simulink model "Modular_Model_New_Board"  (R2016a)
settings: Solver=FixedStepAuto  SolverMode=SingleTasking  StartTime=0.0  StopTime=30e-3  FixedStep=SampleTime*1e-2  MinStep=SampleTime*1e-2  RelTol=1e-3
values from neighbouring files (symbols this model uses):
  ffund = 50    [sim_param_new_board.m]
  ModulationIndex1 = 0.9    [sim_param_new_board.m]
  ModulationIndex2 = 0.9    [sim_param_new_board.m]
  Module1Phase = 0    [sim_param_new_board.m]
  Module2Phase = 180    [sim_param_new_board.m]
  Rin = 10    [sim_param_new_board.m]
  Rload1 = Z1*PF    [sim_param_new_board.m]
  Rload2 = Z2*PF    [sim_param_new_board.m]
  Vmodule = 270    [sim_param_new_board.m]
  VpulseMax = 6    [sim_param_new_board.m]
  VpulseMin = -3    [sim_param_new_board.m]
libraries: elec_lib x139, fl_lib x67, nesl_utility x67, simulink x24, powerlib_meascontrol x4
(part 1 of 4)
settings Model: SimulationMode=accelerator  Creator=Furkan  LastModifiedBy=mesutto
settings DebuggingCC: SFUnexpectedBacktrackingDiag=error  SFNoUnconditionalDefaultTransitionDiag=error
settings GRTTargetCC: TargetLangStandard=C99 (ISO)  GeneratePreprocessorConditionals=Use local settings
settings ConfigComp: CovMetricSettings=dwe  CovHtmlReporting=off  CovSaveCumulativeToWorkspaceVar=off  CovSaveSingleToWorkspaceVar=off  CovExternalEMLEnable=on

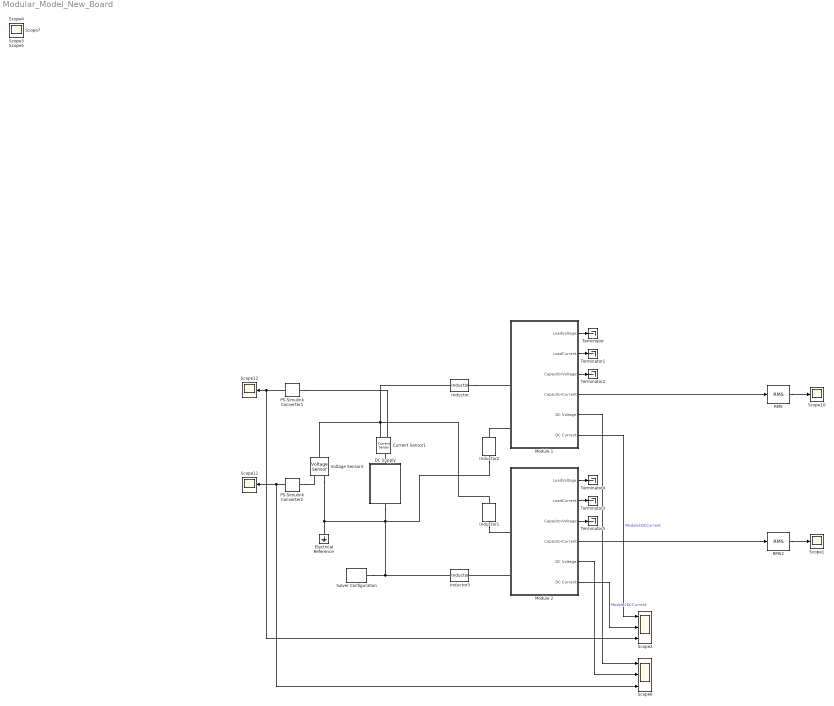
== system Modular_Model_New_Board ==
  Current Sensor1 : fl_lib/Electrical/Electrical Sensors/Current Sensor
  DC Supply : Subsystem
  Electrical Reference : fl_lib/Electrical/Electrical Elements/Electrical Reference
  Inductor : elec_lib/Passive Devices/Inductor  l=POS1 H  L_tol=20  enable_L_tol=0  tol_distribution=1  nSigma=4  r=0 Ohm  g=1e-9 1/Ohm  initI=0 A  enable_operating_limits=0  operating_limit_action=2  max_working_current=1 A  power_rating=1 W  enable_faults=0  fault_action=1  lambdaPercent=50  k_faulted=0.9999  turnsShort=0  openCct=0  groundShort=0  groundShortG=0 1/Ohm  tau_fault=1e-3 s  enable_temporal_fault=0  t_fault=1 s  enable_behavioral_fault=0  max_permissible_voltage=100 V  n_fail_on_voltage=1  max_permissible_current=1 A  t_fail_on_current=1 s
  Inductor1 : elec_lib/Passive Devices/Inductor  l=POS2 H  L_tol=20  enable_L_tol=0  tol_distribution=1  nSigma=4  r=0 Ohm  g=1e-9 1/Ohm  initI=0 A  enable_operating_limits=0  operating_limit_action=2  max_working_current=1 A  power_rating=1 W  enable_faults=0  fault_action=1  lambdaPercent=50  k_faulted=0.9999  turnsShort=0  openCct=0  groundShort=0  groundShortG=0 1/Ohm  tau_fault=1e-3 s  enable_temporal_fault=0  t_fault=1 s  enable_behavioral_fault=0  max_permissible_voltage=100 V  n_fail_on_voltage=1  max_permissible_current=1 A  t_fail_on_current=1 s
  Inductor2 : elec_lib/Passive Devices/Inductor  l=NEG1 H  L_tol=20  enable_L_tol=0  tol_distribution=1  nSigma=4  r=0 Ohm  g=1e-9 1/Ohm  initI=0 A  enable_operating_limits=0  operating_limit_action=2  max_working_current=1 A  power_rating=1 W  enable_faults=0  fault_action=1  lambdaPercent=50  k_faulted=0.9999  turnsShort=0  openCct=0  groundShort=0  groundShortG=0 1/Ohm  tau_fault=1e-3 s  enable_temporal_fault=0  t_fault=1 s  enable_behavioral_fault=0  max_permissible_voltage=100 V  n_fail_on_voltage=1  max_permissible_current=1 A  t_fail_on_current=1 s
  Inductor3 : elec_lib/Passive Devices/Inductor  l=NEG2 H  L_tol=20  enable_L_tol=0  tol_distribution=1  nSigma=4  r=0 Ohm  g=1e-9 1/Ohm  initI=0 A  enable_operating_limits=0  operating_limit_action=2  max_working_current=1 A  power_rating=1 W  enable_faults=0  fault_action=1  lambdaPercent=50  k_faulted=0.9999  turnsShort=0  openCct=0  groundShort=0  groundShortG=0 1/Ohm  tau_fault=1e-3 s  enable_temporal_fault=0  t_fault=1 s  enable_behavioral_fault=0  max_permissible_voltage=100 V  n_fail_on_voltage=1  max_permissible_current=1 A  t_fail_on_current=1 s
  Module 1 : Subsystem
  Module 2 : Subsystem
  PS-Simulink Converter1 : nesl_utility/PS-Simulink Converter  PhysicalDomain=network_engine_domain  SubClassName=ps_output  LeftPortType=input  RightPortType=output  PseudoPeriodic=off  Frequencies=[]  Unit=1  AffineConversion=off
  PS-Simulink Converter2 : nesl_utility/PS-Simulink Converter  PhysicalDomain=network_engine_domain  SubClassName=ps_output  LeftPortType=input  RightPortType=output  PseudoPeriodic=off  Frequencies=[]  Unit=1  AffineConversion=off
  RMS : powerlib_meascontrol/Measurements/RMS  TrueRMS=on  Freq=40000  RMSInit=0  Ts=0
  RMS2 : powerlib_meascontrol/Measurements/RMS  TrueRMS=on  Freq=40000  RMSInit=0  Ts=0
  Scope{1,3..5,7,10..12} (8 alike) : Scope
  Scope2 : Scope  NumInputPorts=3
  Scope6 : Scope  NumInputPorts=3
  Solver Configuration : nesl_utility/Solver Configuration  PhysicalDomain=network_engine_domain  SubClassName=solver  LeftPortType=input  RightPortType=generic  Accelerate=off  Tones=[]  Harmonics=[]  SimulateNoise=off  Profile=off  UseLocalSampling=off  EnableSwitchedLinearOptims=on  FrequencyDomain=off  UseCCode=off  RelTol=0.001  AbsTol=1e-06  MinStep=1e-09  ToWorkspace=off  RevertToSquareIcSolve=off  NumHomotopyIterations=100  PhasorMode=off  PhasorModeNumHarmonics=1  OverrideAbsTol=off  DoDC=off  ResidualTolerance=1e-09  UseLocalSolver=on  LocalSolverChoice=NE_BACKWARD_EULER_ADVANCER  LocalSolverSampleTime=SampleTime  DoFixedCost=on  MaxNonlinIter=3  MaxModeIter=2  LinearAlgebra=Sparse  DelaysMemoryBudget=1024  AutomaticFiltering=on  FilteringTimeConstant=0.001
  Terminator{,1..5} (6 alike) : Terminator
  Voltage Sensor3 : fl_lib/Electrical/Electrical Sensors/Voltage Sensor
  wires:
  Module 1/1(LoadVoltage) -> Terminator/1
  Module 1/4(CapacitorCurrent) -> RMS/1
  Module 2/1(LoadVoltage) -> Terminator4/1
  Module 2/4(CapacitorCurrent) -> RMS2/1
  PS-Simulink Converter2/1 -> Scope6/3, Scope11/1
  PS-Simulink Converter1/1 -> Scope12/1, Scope2/3
  RMS/1 -> Scope10/1
  Module 1/2(LoadCurrent) -> Terminator1/1
  Module 1/3(CapacitorVoltage) -> Terminator2/1
  Module 2/2(LoadCurrent) -> Terminator3/1
  Module 2/3(CapacitorVoltage) -> Terminator5/1
  RMS2/1 -> Scope1/1
  Module 1/6(DC Current) -> Scope2/1  "Module1DCCurrent"
  Module 2/6(DC Current) -> Scope2/2  "Module2DCCurrent"
  Module 1/5(DC Voltage) -> Scope6/1
  Module 2/5(DC Voltage) -> Scope6/2
  connections:
  Inductor1/RConn1 -- Inductor/LConn1 -- Current Sensor1/RConn2 -- Voltage Sensor3/LConn1
  Module 2/LConn3 -- Inductor3/RConn1
  Inductor/RConn1 -- Module 1/LConn2
  Module 1/LConn3 -- Inductor2/RConn1
  Inductor1/LConn1 -- Module 2/LConn2
  PS-Simulink Converter2/LConn1 -- Voltage Sensor3/RConn1
  Electrical Reference/LConn1 -- Inductor2/LConn1 -- DC Supply/LConn1 -- Inductor3/LConn1 -- Solver Configuration/RConn1 -- Voltage Sensor3/RConn2
  Current Sensor1/LConn1 -- DC Supply/RConn1
  PS-Simulink Converter1/LConn1 -- Current Sensor1/RConn1

== system Modular_Model_New_Board/DC Supply ==
  Inductor21 : elec_lib/Passive Devices/Inductor  l=Lin H  L_tol=20  enable_L_tol=0  tol_distribution=1  nSigma=4  r=0 Ohm  g=1e-9 1/Ohm  initI=0 A  enable_operating_limits=0  operating_limit_action=2  max_working_current=1 A  power_rating=1 W  enable_faults=0  fault_action=1  lambdaPercent=50  k_faulted=0.9999  turnsShort=0  openCct=0  groundShort=0  groundShortG=0 1/Ohm  tau_fault=1e-3 s  enable_temporal_fault=0  t_fault=1 s  enable_behavioral_fault=0  max_permissible_voltage=100 V  n_fail_on_voltage=1  max_permissible_current=1 A  t_fail_on_current=1 s
  Resistor18 : elec_lib/Passive Devices/Resistor  R=Rin Ohm  R_tol=5  enable_R_tol=0  tol_distribution=1  nSigma=4  enable_operating_limits=0  operating_limit_action=2  max_working_voltage=100 V  power_rating=1 W  enable_faults=0  fault_action=1  R_faulted=inf Ohm  enable_temporal_fault=0  t_fault=1 s  enable_behavioral_fault=0  max_permissible_current=1 A  t_fail_on_current=1 s  noise_mode=0  sample_time=1e-3 s  repeatability=1  auto_seed=728464307  user_seed=0  Tdevice=25 degC  alpha=3.93e-3 1/K  Tmeas=25 degC  thermal_mass=100 J/K  initial_temperature=25 degC  power_derating_T1=70 degC  power_derating_T2=155 degC  operating_temperature_range_vec=[-50, 150] degC
  Voltage Source : elec_lib/Sources/Voltage Source  dc_voltage=Vin V  ac_voltage=0 V  ac_shift=0 rad  ac_frequency=60 Hz  noise_mode=0  PSD=0 V^2/Hz  sample_time=1e-3 s  repeatability=1  auto_seed=1197368251  user_seed=0
  NEG : PMIOPort  Port=1  Side=Left
  POS : PMIOPort  Port=2  Side=Right
  connections:
  Resistor18/LConn1 -- Voltage Source/LConn1
  Voltage Source/RConn1 -- Inductor21/RConn1
  Inductor21/LConn1 -- NEG/RConn1
  Resistor18/RConn1 -- POS/RConn1

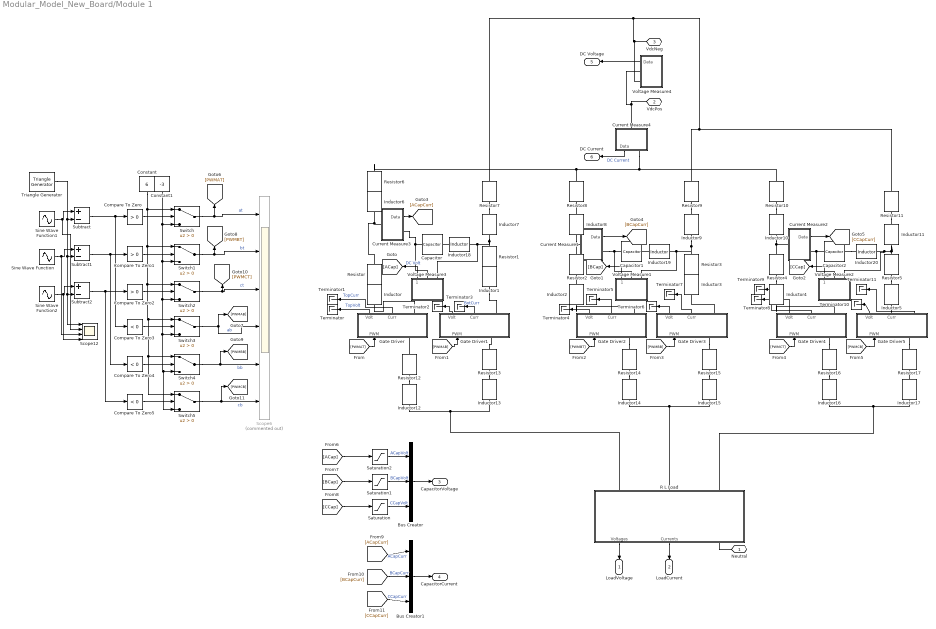
== system Modular_Model_New_Board/Module 1 ==
  Bus Creator : BusCreator  Inputs=3
  Bus Creator1 : BusCreator  Inputs=3
  Capacitor : elec_lib/Passive Devices/Capacitor  enable_table=0  c=C1A F  Cvec=[1e-05, 1e-06] F  Vvec=[0, 10] V  CV_table_symmetry=1  C_tol=0  enable_C_tol=0  tol_distribution=1  nSigma=4  r=21.1e-3 Ohm  g=0 1/Ohm  initV=0 V  enable_operating_limits=0  operating_limit_action=2  max_working_voltage_range=[-25, 25] V  power_rating=1 W  enable_faults=0  fault_action=1  Cscale_faulted=100  R_faulted=1e-3 Ohm  G_faulted=0 1/Ohm  tau_fault=1e-3 s  enable_temporal_fault=0  t_fault=1 s  enable_behavioral_fault=0  max_permissible_voltage_range=[-100, 100] V  t_fail_on_voltage=1 s
  Capacitor1 : elec_lib/Passive Devices/Capacitor  enable_table=0  c=C1B F  Cvec=[1e-05, 1e-06] F  Vvec=[0, 10] V  CV_table_symmetry=1  C_tol=0  enable_C_tol=0  tol_distribution=1  nSigma=4  r=21.1e-3 Ohm  g=0 1/Ohm  initV=0 V  enable_operating_limits=0  operating_limit_action=2  max_working_voltage_range=[-25, 25] V  power_rating=1 W  enable_faults=0  fault_action=1  Cscale_faulted=100  R_faulted=1e-3 Ohm  G_faulted=0 1/Ohm  tau_fault=1e-3 s  enable_temporal_fault=0  t_fault=1 s  enable_behavioral_fault=0  max_permissible_voltage_range=[-100, 100] V  t_fail_on_voltage=1 s
  Capacitor2 : elec_lib/Passive Devices/Capacitor  enable_table=0  c=C1C F  Cvec=[1e-05, 1e-06] F  Vvec=[0, 10] V  CV_table_symmetry=1  C_tol=0  enable_C_tol=0  tol_distribution=1  nSigma=4  r=21.1e-3 Ohm  g=0 1/Ohm  initV=0 V  enable_operating_limits=0  operating_limit_action=2  max_working_voltage_range=[-25, 25] V  power_rating=1 W  enable_faults=0  fault_action=1  Cscale_faulted=100  R_faulted=1e-3 Ohm  G_faulted=0 1/Ohm  tau_fault=1e-3 s  enable_temporal_fault=0  t_fault=1 s  enable_behavioral_fault=0  max_permissible_voltage_range=[-100, 100] V  t_fail_on_voltage=1 s
  Compare To Zero : simulink/Logic and Bit Operations/Compare To Zero  relop=>  OutDataTypeStr=boolean
  Compare To Zero1 : simulink/Logic and Bit Operations/Compare To Zero  relop=>  OutDataTypeStr=boolean
  Compare To Zero2 : simulink/Logic and Bit Operations/Compare To Zero  relop=>  OutDataTypeStr=boolean
  Compare To Zero3 : simulink/Logic and Bit Operations/Compare To Zero  relop=<  OutDataTypeStr=boolean
  Compare To Zero4 : simulink/Logic and Bit Operations/Compare To Zero  relop=<  OutDataTypeStr=boolean
  Compare To Zero5 : simulink/Logic and Bit Operations/Compare To Zero  relop=<  OutDataTypeStr=boolean
  Constant : Constant  Value=6
  Constant1 : Constant  Value=-3
  Current Measure1 : Subsystem
  Current Measure2 : Subsystem
  Current Measure3 : Subsystem
  Current Measure4 : Subsystem
  Gate Driver : Subsystem
  Gate Driver1 : Subsystem
  Gate Driver2 : Subsystem
  Gate Driver3 : Subsystem
  Gate Driver4 : Subsystem
  Gate Driver5 : Subsystem
  Inductor : elec_lib/Passive Devices/Inductor  l=ACapToDrain H  L_tol=20  enable_L_tol=0  tol_distribution=1  nSigma=4  r=0 Ohm  g=1e-9 1/Ohm  initI=0 A  enable_operating_limits=0  operating_limit_action=2  max_working_current=1 A  power_rating=1 W  enable_faults=0  fault_action=1  lambdaPercent=50  k_faulted=0.9999  turnsShort=0  openCct=0  groundShort=0  groundShortG=0 1/Ohm  tau_fault=1e-3 s  enable_temporal_fault=0  t_fault=1 s  enable_behavioral_fault=0  max_permissible_voltage=100 V  n_fail_on_voltage=1  max_permissible_current=1 A  t_fail_on_current=1 s
  Inductor1 : elec_lib/Passive Devices/Inductor  l=ACapToSource H  L_tol=20  enable_L_tol=0  tol_distribution=1  nSigma=4  r=0 Ohm  g=1e-9 1/Ohm  initI=0 A  enable_operating_limits=0  operating_limit_action=2  max_working_current=1 A  power_rating=1 W  enable_faults=0  fault_action=1  lambdaPercent=50  k_faulted=0.9999  turnsShort=0  openCct=0  groundShort=0  groundShortG=0 1/Ohm  tau_fault=1e-3 s  enable_temporal_fault=0  t_fault=1 s  enable_behavioral_fault=0  max_permissible_voltage=100 V  n_fail_on_voltage=1  max_permissible_current=1 A  t_fail_on_current=1 s
  Inductor10 : elec_lib/Passive Devices/Inductor  l=CPosToCap H  L_tol=20  enable_L_tol=0  tol_distribution=1  nSigma=4  r=0 Ohm  g=1e-9 1/Ohm  initI=0 A  enable_operating_limits=0  operating_limit_action=2  max_working_current=1 A  power_rating=1 W  enable_faults=0  fault_action=1  lambdaPercent=50  k_faulted=0.9999  turnsShort=0  openCct=0  groundShort=0  groundShortG=0 1/Ohm  tau_fault=1e-3 s  enable_temporal_fault=0  t_fault=1 s  enable_behavioral_fault=0  max_permissible_voltage=100 V  n_fail_on_voltage=1  max_permissible_current=1 A  t_fail_on_current=1 s
  Inductor11 : elec_lib/Passive Devices/Inductor  l=CNegToCap H  L_tol=20  enable_L_tol=0  tol_distribution=1  nSigma=4  r=0 Ohm  g=1e-9 1/Ohm  initI=0 A  enable_operating_limits=0  operating_limit_action=2  max_working_current=1 A  power_rating=1 W  enable_faults=0  fault_action=1  lambdaPercent=50  k_faulted=0.9999  turnsShort=0  openCct=0  groundShort=0  groundShortG=0 1/Ohm  tau_fault=1e-3 s  enable_temporal_fault=0  t_fault=1 s  enable_behavioral_fault=0  max_permissible_voltage=100 V  n_fail_on_voltage=1  max_permissible_current=1 A  t_fail_on_current=1 s
  Inductor12 : elec_lib/Passive Devices/Inductor  l=ASourceToLoad H  L_tol=20  enable_L_tol=0  tol_distribution=1  nSigma=4  r=0 Ohm  g=1e-9 1/Ohm  initI=0 A  enable_operating_limits=0  operating_limit_action=2  max_working_current=1 A  power_rating=1 W  enable_faults=0  fault_action=1  lambdaPercent=50  k_faulted=0.9999  turnsShort=0  openCct=0  groundShort=0  groundShortG=0 1/Ohm  tau_fault=1e-3 s  enable_temporal_fault=0  t_fault=1 s  enable_behavioral_fault=0  max_permissible_voltage=100 V  n_fail_on_voltage=1  max_permissible_current=1 A  t_fail_on_current=1 s
  Inductor13 : elec_lib/Passive Devices/Inductor  l=ADrainToLoad H  L_tol=20  enable_L_tol=0  tol_distribution=1  nSigma=4  r=0 Ohm  g=1e-9 1/Ohm  initI=0 A  enable_operating_limits=0  operating_limit_action=2  max_working_current=1 A  power_rating=1 W  enable_faults=0  fault_action=1  lambdaPercent=50  k_faulted=0.9999  turnsShort=0  openCct=0  groundShort=0  groundShortG=0 1/Ohm  tau_fault=1e-3 s  enable_temporal_fault=0  t_fault=1 s  enable_behavioral_fault=0  max_permissible_voltage=100 V  n_fail_on_voltage=1  max_permissible_current=1 A  t_fail_on_current=1 s
  Inductor14 : elec_lib/Passive Devices/Inductor  l=BSourceToLoad H  L_tol=20  enable_L_tol=0  tol_distribution=1  nSigma=4  r=0 Ohm  g=1e-9 1/Ohm  initI=0 A  enable_operating_limits=0  operating_limit_action=2  max_working_current=1 A  power_rating=1 W  enable_faults=0  fault_action=1  lambdaPercent=50  k_faulted=0.9999  turnsShort=0  openCct=0  groundShort=0  groundShortG=0 1/Ohm  tau_fault=1e-3 s  enable_temporal_fault=0  t_fault=1 s  enable_behavioral_fault=0  max_permissible_voltage=100 V  n_fail_on_voltage=1  max_permissible_current=1 A  t_fail_on_current=1 s
  Inductor15 : elec_lib/Passive Devices/Inductor  l=BDrainToLoad H  L_tol=20  enable_L_tol=0  tol_distribution=1  nSigma=4  r=0 Ohm  g=1e-9 1/Ohm  initI=0 A  enable_operating_limits=0  operating_limit_action=2  max_working_current=1 A  power_rating=1 W  enable_faults=0  fault_action=1  lambdaPercent=50  k_faulted=0.9999  turnsShort=0  openCct=0  groundShort=0  groundShortG=0 1/Ohm  tau_fault=1e-3 s  enable_temporal_fault=0  t_fault=1 s  enable_behavioral_fault=0  max_permissible_voltage=100 V  n_fail_on_voltage=1  max_permissible_current=1 A  t_fail_on_current=1 s
  Inductor16 : elec_lib/Passive Devices/Inductor  l=CSourceToLoad H  L_tol=20  enable_L_tol=0  tol_distribution=1  nSigma=4  r=0 Ohm  g=1e-9 1/Ohm  initI=0 A  enable_operating_limits=0  operating_limit_action=2  max_working_current=1 A  power_rating=1 W  enable_faults=0  fault_action=1  lambdaPercent=50  k_faulted=0.9999  turnsShort=0  openCct=0  groundShort=0  groundShortG=0 1/Ohm  tau_fault=1e-3 s  enable_temporal_fault=0  t_fault=1 s  enable_behavioral_fault=0  max_permissible_voltage=100 V  n_fail_on_voltage=1  max_permissible_current=1 A  t_fail_on_current=1 s
  Inductor17 : elec_lib/Passive Devices/Inductor  l=CDrainToLoad H  L_tol=20  enable_L_tol=0  tol_distribution=1  nSigma=4  r=0 Ohm  g=1e-9 1/Ohm  initI=0 A  enable_operating_limits=0  operating_limit_action=2  max_working_current=1 A  power_rating=1 W  enable_faults=0  fault_action=1  lambdaPercent=50  k_faulted=0.9999  turnsShort=0  openCct=0  groundShort=0  groundShortG=0 1/Ohm  tau_fault=1e-3 s  enable_temporal_fault=0  t_fault=1 s  enable_behavioral_fault=0  max_permissible_voltage=100 V  n_fail_on_voltage=1  max_permissible_current=1 A  t_fail_on_current=1 s
  Inductor18 : elec_lib/Passive Devices/Inductor  l=19e-9 H  L_tol=20  enable_L_tol=0  tol_distribution=1  nSigma=4  r=0 Ohm  g=1e-9 1/Ohm  initI=0 A  enable_operating_limits=0  operating_limit_action=2  max_working_current=1 A  power_rating=1 W  enable_faults=0  fault_action=1  lambdaPercent=50  k_faulted=0.9999  turnsShort=0  openCct=0  groundShort=0  groundShortG=0 1/Ohm  tau_fault=1e-3 s  enable_temporal_fault=0  t_fault=1 s  enable_behavioral_fault=0  max_permissible_voltage=100 V  n_fail_on_voltage=1  max_permissible_current=1 A  t_fail_on_current=1 s
  Inductor19 : elec_lib/Passive Devices/Inductor  l=19e-9 H  L_tol=20  enable_L_tol=0  tol_distribution=1  nSigma=4  r=0 Ohm  g=1e-9 1/Ohm  initI=0 A  enable_operating_limits=0  operating_limit_action=2  max_working_current=1 A  power_rating=1 W  enable_faults=0  fault_action=1  lambdaPercent=50  k_faulted=0.9999  turnsShort=0  openCct=0  groundShort=0  groundShortG=0 1/Ohm  tau_fault=1e-3 s  enable_temporal_fault=0  t_fault=1 s  enable_behavioral_fault=0  max_permissible_voltage=100 V  n_fail_on_voltage=1  max_permissible_current=1 A  t_fail_on_current=1 s
  Inductor2 : elec_lib/Passive Devices/Inductor  l=BCapToDrain H  L_tol=20  enable_L_tol=0  tol_distribution=1  nSigma=4  r=0 Ohm  g=1e-9 1/Ohm  initI=0 A  enable_operating_limits=0  operating_limit_action=2  max_working_current=1 A  power_rating=1 W  enable_faults=0  fault_action=1  lambdaPercent=50  k_faulted=0.9999  turnsShort=0  openCct=0  groundShort=0  groundShortG=0 1/Ohm  tau_fault=1e-3 s  enable_temporal_fault=0  t_fault=1 s  enable_behavioral_fault=0  max_permissible_voltage=100 V  n_fail_on_voltage=1  max_permissible_current=1 A  t_fail_on_current=1 s
  Inductor20 : elec_lib/Passive Devices/Inductor  l=19e-9 H  L_tol=20  enable_L_tol=0  tol_distribution=1  nSigma=4  r=0 Ohm  g=1e-9 1/Ohm  initI=0 A  enable_operating_limits=0  operating_limit_action=2  max_working_current=1 A  power_rating=1 W  enable_faults=0  fault_action=1  lambdaPercent=50  k_faulted=0.9999  turnsShort=0  openCct=0  groundShort=0  groundShortG=0 1/Ohm  tau_fault=1e-3 s  enable_temporal_fault=0  t_fault=1 s  enable_behavioral_fault=0  max_permissible_voltage=100 V  n_fail_on_voltage=1  max_permissible_current=1 A  t_fail_on_current=1 s
  Inductor3 : elec_lib/Passive Devices/Inductor  l=BCapToSource H  L_tol=20  enable_L_tol=0  tol_distribution=1  nSigma=4  r=0 Ohm  g=1e-9 1/Ohm  initI=0 A  enable_operating_limits=0  operating_limit_action=2  max_working_current=1 A  power_rating=1 W  enable_faults=0  fault_action=1  lambdaPercent=50  k_faulted=0.9999  turnsShort=0  openCct=0  groundShort=0  groundShortG=0 1/Ohm  tau_fault=1e-3 s  enable_temporal_fault=0  t_fault=1 s  enable_behavioral_fault=0  max_permissible_voltage=100 V  n_fail_on_voltage=1  max_permissible_current=1 A  t_fail_on_current=1 s
  Inductor4 : elec_lib/Passive Devices/Inductor  l=CCapToDrain H  L_tol=20  enable_L_tol=0  tol_distribution=1  nSigma=4  r=0 Ohm  g=1e-9 1/Ohm  initI=0 A  enable_operating_limits=0  operating_limit_action=2  max_working_current=1 A  power_rating=1 W  enable_faults=0  fault_action=1  lambdaPercent=50  k_faulted=0.9999  turnsShort=0  openCct=0  groundShort=0  groundShortG=0 1/Ohm  tau_fault=1e-3 s  enable_temporal_fault=0  t_fault=1 s  enable_behavioral_fault=0  max_permissible_voltage=100 V  n_fail_on_voltage=1  max_permissible_current=1 A  t_fail_on_current=1 s
  Inductor5 : elec_lib/Passive Devices/Inductor  l=CCapToSource H  L_tol=20  enable_L_tol=0  tol_distribution=1  nSigma=4  r=0 Ohm  g=1e-9 1/Ohm  initI=0 A  enable_operating_limits=0  operating_limit_action=2  max_working_current=1 A  power_rating=1 W  enable_faults=0  fault_action=1  lambdaPercent=50  k_faulted=0.9999  turnsShort=0  openCct=0  groundShort=0  groundShortG=0 1/Ohm  tau_fault=1e-3 s  enable_temporal_fault=0  t_fault=1 s  enable_behavioral_fault=0  max_permissible_voltage=100 V  n_fail_on_voltage=1  max_permissible_current=1 A  t_fail_on_current=1 s
  Inductor6 : elec_lib/Passive Devices/Inductor  l=APosToCap H  L_tol=20  enable_L_tol=0  tol_distribution=1  nSigma=4  r=0 Ohm  g=1e-9 1/Ohm  initI=0 A  enable_operating_limits=0  operating_limit_action=2  max_working_current=1 A  power_rating=1 W  enable_faults=0  fault_action=1  lambdaPercent=50  k_faulted=0.9999  turnsShort=0  openCct=0  groundShort=0  groundShortG=0 1/Ohm  tau_fault=1e-3 s  enable_temporal_fault=0  t_fault=1 s  enable_behavioral_fault=0  max_permissible_voltage=100 V  n_fail_on_voltage=1  max_permissible_current=1 A  t_fail_on_current=1 s
  Inductor7 : elec_lib/Passive Devices/Inductor  l=ANegToCap H  L_tol=20  enable_L_tol=0  tol_distribution=1  nSigma=4  r=0 Ohm  g=1e-9 1/Ohm  initI=0 A  enable_operating_limits=0  operating_limit_action=2  max_working_current=1 A  power_rating=1 W  enable_faults=0  fault_action=1  lambdaPercent=50  k_faulted=0.9999  turnsShort=0  openCct=0  groundShort=0  groundShortG=0 1/Ohm  tau_fault=1e-3 s  enable_temporal_fault=0  t_fault=1 s  enable_behavioral_fault=0  max_permissible_voltage=100 V  n_fail_on_voltage=1  max_permissible_current=1 A  t_fail_on_current=1 s
  Inductor8 : elec_lib/Passive Devices/Inductor  l=BPosToCap H  L_tol=20  enable_L_tol=0  tol_distribution=1  nSigma=4  r=0 Ohm  g=1e-9 1/Ohm  initI=0 A  enable_operating_limits=0  operating_limit_action=2  max_working_current=1 A  power_rating=1 W  enable_faults=0  fault_action=1  lambdaPercent=50  k_faulted=0.9999  turnsShort=0  openCct=0  groundShort=0  groundShortG=0 1/Ohm  tau_fault=1e-3 s  enable_temporal_fault=0  t_fault=1 s  enable_behavioral_fault=0  max_permissible_voltage=100 V  n_fail_on_voltage=1  max_permissible_current=1 A  t_fail_on_current=1 s
  Inductor9 : elec_lib/Passive Devices/Inductor  l=BNegToCap H  L_tol=20  enable_L_tol=0  tol_distribution=1  nSigma=4  r=0 Ohm  g=1e-9 1/Ohm  initI=0 A  enable_operating_limits=0  operating_limit_action=2  max_working_current=1 A  power_rating=1 W  enable_faults=0  fault_action=1  lambdaPercent=50  k_faulted=0.9999  turnsShort=0  openCct=0  groundShort=0  groundShortG=0 1/Ohm  tau_fault=1e-3 s  enable_temporal_fault=0  t_fault=1 s  enable_behavioral_fault=0  max_permissible_voltage=100 V  n_fail_on_voltage=1  max_permissible_current=1 A  t_fail_on_current=1 s
  R L Load : Subsystem
  Resistor : elec_lib/Passive Devices/Resistor  R=854e-6 Ohm  R_tol=5  enable_R_tol=0  tol_distribution=1  nSigma=4  enable_operating_limits=0  operating_limit_action=2  max_working_voltage=100 V  power_rating=1 W  enable_faults=0  fault_action=1  R_faulted=inf Ohm  enable_temporal_fault=0  t_fault=1 s  enable_behavioral_fault=0  max_permissible_current=1 A  t_fail_on_current=1 s  noise_mode=0  sample_time=1e-3 s  repeatability=1  auto_seed=1725752364  user_seed=0  Tdevice=25 degC  alpha=3.93e-3 1/K  Tmeas=25 degC  thermal_mass=100 J/K  initial_temperature=25 degC  power_derating_T1=70 degC  power_derating_T2=155 degC  operating_temperature_range_vec=[-50, 150] degC
  Resistor1 : elec_lib/Passive Devices/Resistor  R=664e-6 Ohm  R_tol=5  enable_R_tol=0  tol_distribution=1  nSigma=4  enable_operating_limits=0  operating_limit_action=2  max_working_voltage=100 V  power_rating=1 W  enable_faults=0  fault_action=1  R_faulted=inf Ohm  enable_temporal_fault=0  t_fault=1 s  enable_behavioral_fault=0  max_permissible_current=1 A  t_fail_on_current=1 s  noise_mode=0  sample_time=1e-3 s  repeatability=1  auto_seed=1978802833  user_seed=0  Tdevice=25 degC  alpha=3.93e-3 1/K  Tmeas=25 degC  thermal_mass=100 J/K  initial_temperature=25 degC  power_derating_T1=70 degC  power_derating_T2=155 degC  operating_temperature_range_vec=[-50, 150] degC
  Resistor10 : elec_lib/Passive Devices/Resistor  R=867e-6 Ohm  R_tol=5  enable_R_tol=0  tol_distribution=1  nSigma=4  enable_operating_limits=0  operating_limit_action=2  max_working_voltage=100 V  power_rating=1 W  enable_faults=0  fault_action=1  R_faulted=inf Ohm  enable_temporal_fault=0  t_fault=1 s  enable_behavioral_fault=0  max_permissible_current=1 A  t_fail_on_current=1 s  noise_mode=0  sample_time=1e-3 s  repeatability=1  auto_seed=3085328168  user_seed=0  Tdevice=25 degC  alpha=3.93e-3 1/K  Tmeas=25 degC  thermal_mass=100 J/K  initial_temperature=25 degC  power_derating_T1=70 degC  power_derating_T2=155 degC  operating_temperature_range_vec=[-50, 150] degC
  Resistor11 : elec_lib/Passive Devices/Resistor  R=595e-6 Ohm  R_tol=5  enable_R_tol=0  tol_distribution=1  nSigma=4  enable_operating_limits=0  operating_limit_action=2  max_working_voltage=100 V  power_rating=1 W  enable_faults=0  fault_action=1  R_faulted=inf Ohm  enable_temporal_fault=0  t_fault=1 s  enable_behavioral_fault=0  max_permissible_current=1 A  t_fail_on_current=1 s  noise_mode=0  sample_time=1e-3 s  repeatability=1  auto_seed=4160317194  user_seed=0  Tdevice=25 degC  alpha=3.93e-3 1/K  Tmeas=25 degC  thermal_mass=100 J/K  initial_temperature=25 degC  power_derating_T1=70 degC  power_derating_T2=155 degC  operating_temperature_range_vec=[-50, 150] degC
  Resistor12 : elec_lib/Passive Devices/Resistor  R=218.8e-6 Ohm  R_tol=5  enable_R_tol=0  tol_distribution=1  nSigma=4  enable_operating_limits=0  operating_limit_action=2  max_working_voltage=100 V  power_rating=1 W  enable_faults=0  fault_action=1  R_faulted=inf Ohm  enable_temporal_fault=0  t_fault=1 s  enable_behavioral_fault=0  max_permissible_current=1 A  t_fail_on_current=1 s  noise_mode=0  sample_time=1e-3 s  repeatability=1  auto_seed=1396490070  user_seed=0  Tdevice=25 degC  alpha=3.93e-3 1/K  Tmeas=25 degC  thermal_mass=100 J/K  initial_temperature=25 degC  power_derating_T1=70 degC  power_derating_T2=155 degC  operating_temperature_range_vec=[-50, 150] degC
  Resistor13 : elec_lib/Passive Devices/Resistor  R=218.8e-6 Ohm  R_tol=5  enable_R_tol=0  tol_distribution=1  nSigma=4  enable_operating_limits=0  operating_limit_action=2  max_working_voltage=100 V  power_rating=1 W  enable_faults=0  fault_action=1  R_faulted=inf Ohm  enable_temporal_fault=0  t_fault=1 s  enable_behavioral_fault=0  max_permissible_current=1 A  t_fail_on_current=1 s  noise_mode=0  sample_time=1e-3 s  repeatability=1  auto_seed=453673974  user_seed=0  Tdevice=25 degC  alpha=3.93e-3 1/K  Tmeas=25 degC  thermal_mass=100 J/K  initial_temperature=25 degC  power_derating_T1=70 degC  power_derating_T2=155 degC  operating_temperature_range_vec=[-50, 150] degC
  Resistor14 : elec_lib/Passive Devices/Resistor  R=218e-6 Ohm  R_tol=5  enable_R_tol=0  tol_distribution=1  nSigma=4  enable_operating_limits=0  operating_limit_action=2  max_working_voltage=100 V  power_rating=1 W  enable_faults=0  fault_action=1  R_faulted=inf Ohm  enable_temporal_fault=0  t_fault=1 s  enable_behavioral_fault=0  max_permissible_current=1 A  t_fail_on_current=1 s  noise_mode=0  sample_time=1e-3 s  repeatability=1  auto_seed=2624047458  user_seed=0  Tdevice=25 degC  alpha=3.93e-3 1/K  Tmeas=25 degC  thermal_mass=100 J/K  initial_temperature=25 degC  power_derating_T1=70 degC  power_derating_T2=155 degC  operating_temperature_range_vec=[-50, 150] degC
  Resistor15 : elec_lib/Passive Devices/Resistor  R=218e-6 Ohm  R_tol=5  enable_R_tol=0  tol_distribution=1  nSigma=4  enable_operating_limits=0  operating_limit_action=2  max_working_voltage=100 V  power_rating=1 W  enable_faults=0  fault_action=1  R_faulted=inf Ohm  enable_temporal_fault=0  t_fault=1 s  enable_behavioral_fault=0  max_permissible_current=1 A  t_fail_on_current=1 s  noise_mode=0  sample_time=1e-3 s  repeatability=1  auto_seed=3344930158  user_seed=0  Tdevice=25 degC  alpha=3.93e-3 1/K  Tmeas=25 degC  thermal_mass=100 J/K  initial_temperature=25 degC  power_derating_T1=70 degC  power_derating_T2=155 degC  operating_temperature_range_vec=[-50, 150] degC
  Resistor16 : elec_lib/Passive Devices/Resistor  R=218.3e-6 Ohm  R_tol=5  enable_R_tol=0  tol_distribution=1  nSigma=4  enable_operating_limits=0  operating_limit_action=2  max_working_voltage=100 V  power_rating=1 W  enable_faults=0  fault_action=1  R_faulted=inf Ohm  enable_temporal_fault=0  t_fault=1 s  enable_behavioral_fault=0  max_permissible_current=1 A  t_fail_on_current=1 s  noise_mode=0  sample_time=1e-3 s  repeatability=1  auto_seed=1818716438  user_seed=0  Tdevice=25 degC  alpha=3.93e-3 1/K  Tmeas=25 degC  thermal_mass=100 J/K  initial_temperature=25 degC  power_derating_T1=70 degC  power_derating_T2=155 degC  operating_temperature_range_vec=[-50, 150] degC
  Resistor17 : elec_lib/Passive Devices/Resistor  R=218.3e-6 Ohm  R_tol=5  enable_R_tol=0  tol_distribution=1  nSigma=4  enable_operating_limits=0  operating_limit_action=2  max_working_voltage=100 V  power_rating=1 W  enable_faults=0  fault_action=1  R_faulted=inf Ohm  enable_temporal_fault=0  t_fault=1 s  enable_behavioral_fault=0  max_permissible_current=1 A  t_fail_on_current=1 s  noise_mode=0  sample_time=1e-3 s  repeatability=1  auto_seed=390083043  user_seed=0  Tdevice=25 degC  alpha=3.93e-3 1/K  Tmeas=25 degC  thermal_mass=100 J/K  initial_temperature=25 degC  power_derating_T1=70 degC  power_derating_T2=155 degC  operating_temperature_range_vec=[-50, 150] degC
  Resistor2 : elec_lib/Passive Devices/Resistor  R=813e-6 Ohm  R_tol=5  enable_R_tol=0  tol_distribution=1  nSigma=4  enable_operating_limits=0  operating_limit_action=2  max_working_voltage=100 V  power_rating=1 W  enable_faults=0  fault_action=1  R_faulted=inf Ohm  enable_temporal_fault=0  t_fault=1 s  enable_behavioral_fault=0  max_permissible_current=1 A  t_fail_on_current=1 s  noise_mode=0  sample_time=1e-3 s  repeatability=1  auto_seed=4216102895  user_seed=0  Tdevice=25 degC  alpha=3.93e-3 1/K  Tmeas=25 degC  thermal_mass=100 J/K  initial_temperature=25 degC  power_derating_T1=70 degC  power_derating_T2=155 degC  operating_temperature_range_vec=[-50, 150] degC
  Resistor3 : elec_lib/Passive Devices/Resistor  R=664e-6 Ohm  R_tol=5  enable_R_tol=0  tol_distribution=1  nSigma=4  enable_operating_limits=0  operating_limit_action=2  max_working_voltage=100 V  power_rating=1 W  enable_faults=0  fault_action=1  R_faulted=inf Ohm  enable_temporal_fault=0  t_fault=1 s  enable_behavioral_fault=0  max_permissible_current=1 A  t_fail_on_current=1 s  noise_mode=0  sample_time=1e-3 s  repeatability=1  auto_seed=671754155  user_seed=0  Tdevice=25 degC  alpha=3.93e-3 1/K  Tmeas=25 degC  thermal_mass=100 J/K  initial_temperature=25 degC  power_derating_T1=70 degC  power_derating_T2=155 degC  operating_temperature_range_vec=[-50, 150] degC
  Resistor4 : elec_lib/Passive Devices/Resistor  R=854e-6 Ohm  R_tol=5  enable_R_tol=0  tol_distribution=1  nSigma=4  enable_operating_limits=0  operating_limit_action=2  max_working_voltage=100 V  power_rating=1 W  enable_faults=0  fault_action=1  R_faulted=inf Ohm  enable_temporal_fault=0  t_fault=1 s  enable_behavioral_fault=0  max_permissible_current=1 A  t_fail_on_current=1 s  noise_mode=0  sample_time=1e-3 s  repeatability=1  auto_seed=3674442472  user_seed=0  Tdevice=25 degC  alpha=3.93e-3 1/K  Tmeas=25 degC  thermal_mass=100 J/K  initial_temperature=25 degC  power_derating_T1=70 degC  power_derating_T2=155 degC  operating_temperature_range_vec=[-50, 150] degC
  Resistor5 : elec_lib/Passive Devices/Resistor  R=664e-6 Ohm  R_tol=5  enable_R_tol=0  tol_distribution=1  nSigma=4  enable_operating_limits=0  operating_limit_action=2  max_working_voltage=100 V  power_rating=1 W  enable_faults=0  fault_action=1  R_faulted=inf Ohm  enable_temporal_fault=0  t_fault=1 s  enable_behavioral_fault=0  max_permissible_current=1 A  t_fail_on_current=1 s  noise_mode=0  sample_time=1e-3 s  repeatability=1  auto_seed=2769242599  user_seed=0  Tdevice=25 degC  alpha=3.93e-3 1/K  Tmeas=25 degC  thermal_mass=100 J/K  initial_temperature=25 degC  power_derating_T1=70 degC  power_derating_T2=155 degC  operating_temperature_range_vec=[-50, 150] degC
  Resistor6 : elec_lib/Passive Devices/Resistor  R=1037e-6 Ohm  R_tol=5  enable_R_tol=0  tol_distribution=1  nSigma=4  enable_operating_limits=0  operating_limit_action=2  max_working_voltage=100 V  power_rating=1 W  enable_faults=0  fault_action=1  R_faulted=inf Ohm  enable_temporal_fault=0  t_fault=1 s  enable_behavioral_fault=0  max_permissible_current=1 A  t_fail_on_current=1 s  noise_mode=0  sample_time=1e-3 s  repeatability=1  auto_seed=2280044724  user_seed=0  Tdevice=25 degC  alpha=3.93e-3 1/K  Tmeas=25 degC  thermal_mass=100 J/K  initial_temperature=25 degC  power_derating_T1=70 degC  power_derating_T2=155 degC  operating_temperature_range_vec=[-50, 150] degC
  Resistor7 : elec_lib/Passive Devices/Resistor  R=1422e-6 Ohm  R_tol=5  enable_R_tol=0  tol_distribution=1  nSigma=4  enable_operating_limits=0  operating_limit_action=2  max_working_voltage=100 V  power_rating=1 W  enable_faults=0  fault_action=1  R_faulted=inf Ohm  enable_temporal_fault=0  t_fault=1 s  enable_behavioral_fault=0  max_permissible_current=1 A  t_fail_on_current=1 s  noise_mode=0  sample_time=1e-3 s  repeatability=1  auto_seed=2810822912  user_seed=0  Tdevice=25 degC  alpha=3.93e-3 1/K  Tmeas=25 degC  thermal_mass=100 J/K  initial_temperature=25 degC  power_derating_T1=70 degC  power_derating_T2=155 degC  operating_temperature_range_vec=[-50, 150] degC
  Resistor8 : elec_lib/Passive Devices/Resistor  R=611e-6 Ohm  R_tol=5  enable_R_tol=0  tol_distribution=1  nSigma=4  enable_operating_limits=0  operating_limit_action=2  max_working_voltage=100 V  power_rating=1 W  enable_faults=0  fault_action=1  R_faulted=inf Ohm  enable_temporal_fault=0  t_fault=1 s  enable_behavioral_fault=0  max_permissible_current=1 A  t_fail_on_current=1 s  noise_mode=0  sample_time=1e-3 s  repeatability=1  auto_seed=1750711121  user_seed=0  Tdevice=25 degC  alpha=3.93e-3 1/K  Tmeas=25 degC  thermal_mass=100 J/K  initial_temperature=25 degC  power_derating_T1=70 degC  power_derating_T2=155 degC  operating_temperature_range_vec=[-50, 150] degC
  Resistor9 : elec_lib/Passive Devices/Resistor  R=662e-6 Ohm  R_tol=5  enable_R_tol=0  tol_distribution=1  nSigma=4  enable_operating_limits=0  operating_limit_action=2  max_working_voltage=100 V  power_rating=1 W  enable_faults=0  fault_action=1  R_faulted=inf Ohm  enable_temporal_fault=0  t_fault=1 s  enable_behavioral_fault=0  max_permissible_current=1 A  t_fail_on_current=1 s  noise_mode=0  sample_time=1e-3 s  repeatability=1  auto_seed=3521792535  user_seed=0  Tdevice=25 degC  alpha=3.93e-3 1/K  Tmeas=25 degC  thermal_mass=100 J/K  initial_temperature=25 degC  power_derating_T1=70 degC  power_derating_T2=155 degC  operating_temperature_range_vec=[-50, 150] degC
  Saturation : Saturate  UpperLimit=Vmodule*1.5  LowerLimit=-20
  Saturation1 : Saturate  UpperLimit=Vmodule*1.5  LowerLimit=-20
  Saturation2 : Saturate  UpperLimit=Vmodule*1.5  LowerLimit=-20
  Scope12 : Scope  NumInputPorts=4
  Scope6 : Scope  Commented=on  NumInputPorts=6
  Sine Wave Function : Sin  Amplitude=ModulationIndex1  Frequency=ffund*2*pi  Phase=-2*pi/3  SampleTime=0
  Sine Wave Function1 : Sin  Amplitude=ModulationIndex1  Frequency=ffund*2*pi  SampleTime=0
  Sine Wave Function2 : Sin  Amplitude=ModulationIndex1  Frequency=ffund*2*pi  Phase=2*pi/3  SampleTime=0
  Subtract : Sum  Inputs=+-
  Subtract1 : Sum  Inputs=+-
  Subtract2 : Sum  Inputs=+-
  Switch{,1..5} (6 alike) : Switch  Criteria=u2 > Threshold
  Terminator{,1..11} (12 alike) : Terminator
  Triangle Generator : powerlib_meascontrol/Pulse & Signal Generators/Triangle Generator  Freq=fsw  Phase=Module1Phase  Ts=0
  Voltage Measure1 : Subsystem
  Voltage Measure2 : Subsystem
  Voltage Measure3 : Subsystem
  Voltage Measure4 : Subsystem
  "Neutral " : PMIOPort  Port=1  Side=Left
  VdcPos : PMIOPort  Port=2  Side=Left
  VdcNeg : PMIOPort  Port=3  Side=Left
  LoadVoltage : Outport
  LoadCurrent : Outport  Port=2
  CapacitorVoltage : Outport  Port=3
  CapacitorCurrent : Outport  Port=4
  DC Voltage : Outport  Port=5
  DC Current : Outport  Port=6
  wires:
  Compare To Zero3/1 -> Switch3/2
  Switch5/1 -> [PWMCB], Scope6/6  "cb"
  R L Load/2(Currents) -> LoadCurrent/1
  Compare To Zero/1 -> Switch/2
  Subtract2/1 -> Compare To Zero5/1, Compare To Zero2/1
  Constant1/1 -> Switch/3, Switch1/3, Switch5/3, Switch4/3, Switch3/3, Switch2/3
  Gate Driver2/2(Curr) -> Terminator5/1
  Switch/1 -> [PWMAT], Scope6/1  "at"
  Compare To Zero1/1 -> Switch1/2
  Subtract/1 -> Compare To Zero3/1, Compare To Zero/1
  Compare To Zero2/1 -> Switch2/2
  Voltage Measure1/1(Data) -> [BCap]
  [PWMAT] -> Gate Driver/1(PWM)
  Gate Driver3/1(Volt) -> Terminator6/1
  Switch4/1 -> [PWMBB], Scope6/5  "bb"
  Voltage Measure2/1(Data) -> [CCap]
  [PWMBB] -> Gate Driver3/1(PWM)
  Switch3/1 -> [PWMAB], Scope6/4  "ab"
  [PWMAB] -> Gate Driver1/1(PWM)
  Current Measure1/1(Data) -> [BCapCurr]
  Sine Wave Function1/1 -> Scope12/2, Subtract/1
  Constant/1 -> Switch5/1, Switch4/1, Switch3/1, Switch2/1, Switch1/1, Switch/1
  Triangle Generator/1 -> Scope12/1, Subtract2/2, Subtract1/2, Subtract/2
  Voltage Measure3/1(Data) -> [ACap]  "DC Volt"
  Sine Wave Function/1 -> Subtract1/1, Scope12/3
  [PWMCB] -> Gate Driver5/1(PWM)
  [PWMBT] -> Gate Driver2/1(PWM)
  Compare To Zero4/1 -> Switch4/2
  R L Load/1(Voltages) -> LoadVoltage/1
  Gate Driver/1(Volt) -> Terminator/1  "TopVolt"
  Gate Driver1/1(Volt) -> Terminator2/1
  Gate Driver4/1(Volt) -> Terminator8/1
  Gate Driver1/2(Curr) -> Terminator3/1  "BotCurr"
  Subtract1/1 -> Compare To Zero4/1, Compare To Zero1/1
  Gate Driver3/2(Curr) -> Terminator7/1
  Gate Driver4/2(Curr) -> Terminator9/1
  Gate Driver5/1(Volt) -> Terminator10/1
  Sine Wave Function2/1 -> Scope12/4, Subtract2/1
  Gate Driver5/2(Curr) -> Terminator11/1
  Current Measure3/1(Data) -> [ACapCurr]
  Current Measure2/1(Data) -> [CCapCurr]
  Switch1/1 -> [PWMBT], Scope6/2  "bt"
  [PWMCT] -> Gate Driver4/1(PWM)
  Compare To Zero5/1 -> Switch5/2
  Switch2/1 -> [PWMCT], Scope6/3  "ct"
  Gate Driver2/1(Volt) -> Terminator4/1
  Gate Driver/2(Curr) -> Terminator1/1  "TopCurr"
  [ACap] -> Saturation2/1
  [BCap] -> Saturation1/1
  [CCap] -> Saturation/1
  Bus Creator/1 -> CapacitorVoltage/1
  [CCapCurr] -> Bus Creator1/3  "CCapCurr"
  [BCapCurr] -> Bus Creator1/2  "BCapCurr"
  [ACapCurr] -> Bus Creator1/1  "ACapCurr"
  Bus Creator1/1 -> CapacitorCurrent/1
  Current Measure4/1(Data) -> DC Current/1  "DC Current"
  Voltage Measure4/1(Data) -> DC Voltage/1
  Saturation/1 -> Bus Creator/3  "CCapVolt"
  Saturation1/1 -> Bus Creator/2  "BCapVolt"
  Saturation2/1 -> Bus Creator/1  "ACapVolt"
  connections:
  Gate Driver4/LConn1 -- Resistor16/RConn1
  Voltage Measure3/RConn1 -- Current Measure3/RConn1 -- Capacitor/LConn1
  Inductor/LConn1 -- Gate Driver/RConn1
  Resistor3/LConn1 -- Inductor3/RConn1
  Capacitor2/RConn1 -- Inductor20/LConn1
  Gate Driver3/RConn1 -- Inductor3/LConn1
  Inductor14/LConn1 -- R L Load/LConn2 -- Inductor15/LConn1
  Resistor6/RConn1 -- Current Measure4/RConn1 -- Resistor10/RConn1 -- Resistor8/RConn1
  Resistor12/LConn1 -- Inductor12/RConn1
  Inductor4/LConn1 -- Gate Driver4/RConn1
  Inductor16/LConn1 -- R L Load/LConn3 -- Inductor17/LConn1
  Inductor12/LConn1 -- R L Load/LConn1 -- Inductor13/LConn1
  Voltage Measure1/RConn1 -- Capacitor1/LConn1 -- Current Measure1/RConn1
  Resistor4/LConn1 -- Inductor4/RConn1
  Resistor1/RConn1 -- Voltage Measure3/RConn2 -- Inductor18/RConn1 -- Inductor7/LConn1
  Resistor7/RConn1 -- Voltage Measure4/RConn2 -- VdcNeg/RConn1 -- Resistor11/RConn1 -- Resistor9/RConn1
  Gate Driver2/LConn1 -- Resistor14/RConn1
  Resistor12/RConn1 -- Gate Driver/LConn1
  Resistor9/LConn1 -- Inductor9/RConn1
  Resistor13/LConn1 -- Inductor13/RConn1
  Resistor15/LConn1 -- Inductor15/RConn1
  Inductor20/RConn1 -- Voltage Measure2/RConn2 -- Resistor5/RConn1 -- Inductor11/LConn1
  Inductor8/RConn1 -- Resistor8/LConn1
  Inductor6/RConn1 -- Resistor6/LConn1
  Voltage Measure2/RConn1 -- Capacitor2/LConn1 -- Current Measure2/RConn1
  Inductor8/LConn1 -- Current Measure1/LConn1 -- Resistor2/RConn1
  Resistor3/RConn1 -- Voltage Measure1/RConn2 -- Inductor19/RConn1 -- Inductor9/LConn1
  Inductor/RConn1 -- Resistor/LConn1
  Inductor2/RConn1 -- Resistor2/LConn1
  Resistor7/LConn1 -- Inductor7/RConn1
  Resistor14/LConn1 -- Inductor14/RConn1
  Gate Driver3/LConn1 -- Resistor15/RConn1
  Inductor1/LConn1 -- Gate Driver1/RConn1
  Resistor1/LConn1 -- Inductor1/RConn1
  Current Measure3/LConn1 -- Resistor/RConn1 -- Inductor6/LConn1
  Inductor17/RConn1 -- Resistor17/LConn1
  Inductor2/LConn1 -- Gate Driver2/RConn1
  Gate Driver1/LConn1 -- Resistor13/RConn1
  Inductor5/LConn1 -- Gate Driver5/RConn1
  Resistor11/LConn1 -- Inductor11/RConn1
  Resistor16/LConn1 -- Inductor16/RConn1
  Gate Driver5/LConn1 -- Resistor17/RConn1
  Resistor10/LConn1 -- Inductor10/RConn1
  Inductor18/LConn1 -- Capacitor/RConn1
  Capacitor1/RConn1 -- Inductor19/LConn1
  Inductor10/LConn1 -- Current Measure2/LConn1 -- Resistor4/RConn1
  Resistor5/LConn1 -- Inductor5/RConn1
  R L Load/RConn1 -- "Neutral "/RConn1
  Current Measure4/LConn1 -- Voltage Measure4/RConn1 -- VdcPos/RConn1
